simulink model "UAV_Model_template"  (R2025b)
settings: Solver=VariableStepAuto  StartTime=0.0  StopTime=50  FixedStep=Step_Size  RelTol=1e-3  EnableMultiTasking=on
values from neighbouring files (symbols this model uses):
  Init_Pos = [ 0.0, 0.0, -100.0 ]    [main_E2.m]
  Init_Rate = [ x_trim(4), x_trim(5), x_trim(6) ]    [main_E2.m]
  Init_Vel = [ x_trim(1), x_trim(2), x_trim(3) ]    [main_E2.m]
  K_p = 1    [model_data.mat]
  K_q = 3    [model_data.mat]
  K_r = -1    [model_data.mat]
  K_roll = 3    [model_data.mat]
  K_theta = 4    [model_data.mat]
  K_vt = 5    [model_data.mat]
  Max_del_a = 0.523598775598    [model_data.mat]
  Max_del_e = 0.523598775598    [model_data.mat]
  Max_del_r = 0.523598775598    [model_data.mat]
  Max_del_T = 10    [model_data.mat]
  tau_a = 0.5    [model_data.mat]
  tau_e = 0.5    [model_data.mat]
  tau_r = 0.5    [model_data.mat]
  tau_T = 0.2    [model_data.mat]
  u_trim = [0.186847387435 -0.168691706131 2.20732861993e-24 8.61178457979e-24]    [model_data.mat]
  UNIT_GRAV = 9.81    [main_E2.m]
  x_trim = [19.7714170486 1.55747135078e-22 3.01513977975 3.57452064707e-26 1.12807765409e-24 6.034407576e-27 1.79365250696e-25 0.151333968898 -1.40042455829e-45 -2.75841298622e-46 3.7376372575e-41 -5.9107417756e-40]    [model_data.mat]
libraries: UAV_Model_library x16, aerolibconvert2 x3, shared6dofsys x1, aerolibtransform2 x1, matrix_library x1, sharedutil x1, shared6dof x1
settings Model: Creator=e803534  LastModifiedBy=82104
settings SolverCC: AlgebraicLoopSolver=TrustRegion
settings DataIOCC: ReturnWorkspaceOutputs=off
settings OptimizationCC: LifeSpan=inf
settings DebuggingCC: UnconnectedInputMsg=warning  UnconnectedOutputMsg=warning  UnconnectedLineMsg=warning  SFUnexpectedBacktrackingDiag=warning  SFNoUnconditionalDefaultTransitionDiag=warning  ArithmeticOperatorsInVariantConditions=warning
settings ModelReferenceCC: EnableRefExpFcnMdlSchedulingChecks=on
settings SFSimCC: SimUseLocalCustomCode=off  CustomCodeUndefinedFunction=UseInterfaceOnly
settings RTWCC: RTWUseLocalCustomCode=off  GPUComputeCapability=3.5
settings CodeAppCC: StateflowObjectComments=on
settings GRTTargetCC: TargetLangStandard=C89/C90 (ANSI)
settings ConfigComp: CovMetricSettings=dw  CovSaveCumulativeToWorkspaceVar=on  CovSaveSingleToWorkspaceVar=on  CovExternalEMLEnable=off

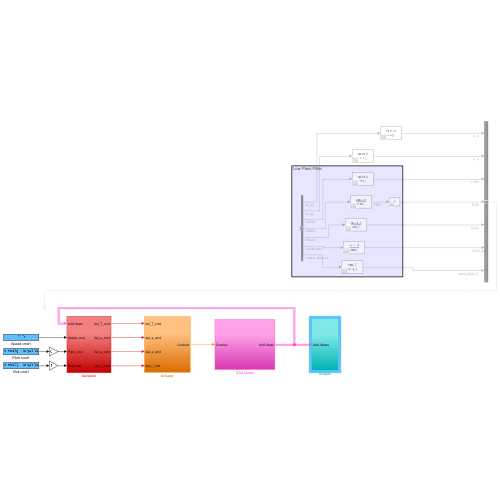
[thumbnail: Simulink's stored preview of the top-level diagram]
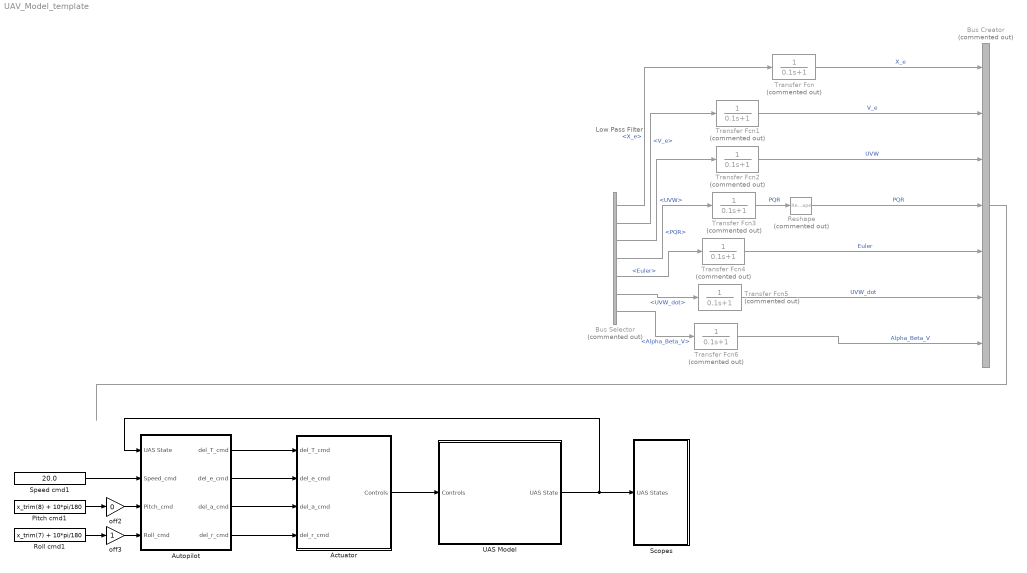
== system UAV_Model_template ==
  note: Low Pass Filter
  Actuator : Subsystem
  Autopilot : Subsystem
  Bus Creator : BusCreator  Commented=on  Inputs=7
  Bus Selector : BusSelector  Commented=on  OutputSignals=X_e,V_e,UVW,PQR,Euler,UVW_dot,Alpha_Beta_V
  Pitch cmd1 : Constant  Value=x_trim(8) + 10*pi/180
  Reshape : Reshape  Commented=on  OutputDimensionality=Customize  OutputDimensions=[3,1]
  Roll cmd1 : Constant  Value=x_trim(7) + 10*pi/180
  Scopes : Subsystem
  Speed cmd1 : Constant  Value=20.0
  Transfer Fcn{,1..6} (7 alike) : TransferFcn  Commented=on  Denominator=[0.1 1]
  UAS Model : Subsystem
  off2 : Gain  Gain=0
  off3 : Gain
  wires:
  Speed cmd1/1 -> Autopilot/2(Speed_cmd)
  Autopilot/1(del_T_cmd) -> Actuator/1(del_T_cmd)
  Autopilot/2(del_e_cmd) -> Actuator/2(del_e_cmd)
  Autopilot/4(del_r_cmd) -> Actuator/4(del_r_cmd)
  Autopilot/3(del_a_cmd) -> Actuator/3(del_a_cmd)
  off2/1 -> Autopilot/3(Pitch_cmd)
  Pitch cmd1/1 -> off2/1
  off3/1 -> Autopilot/4(Roll_cmd)
  Roll cmd1/1 -> off3/1
  UAS Model/1(UAS State) -> Autopilot/1(UAS State), Scopes/1(UAS States)
  Actuator/1(Controls) -> UAS Model/1(Controls)
  Bus Selector/1 -> Transfer Fcn/1  "<X_e>"
  Bus Selector/2 -> Transfer Fcn1/1  "<V_e>"
  Bus Selector/3 -> Transfer Fcn2/1  "<UVW>"
  Bus Selector/4 -> Transfer Fcn3/1  "<PQR>"
  Bus Selector/5 -> Transfer Fcn4/1  "<Euler>"
  Bus Selector/6 -> Transfer Fcn5/1  "<UVW_dot>"
  Bus Selector/7 -> Transfer Fcn6/1  "<Alpha_Beta_V>"
  Transfer Fcn/1 -> Bus Creator/1  "X_e"
  Reshape/1 -> Bus Creator/4  "PQR"
  Transfer Fcn1/1 -> Bus Creator/2  "V_e"
  Transfer Fcn5/1 -> Bus Creator/6  "UVW_dot"
  Transfer Fcn4/1 -> Bus Creator/5  "Euler"
  Transfer Fcn6/1 -> Bus Creator/7  "Alpha_Beta_V"
  Transfer Fcn2/1 -> Bus Creator/3  "UVW"
  Bus Creator/1 -> ?
  Transfer Fcn3/1 -> Reshape/1  "PQR"

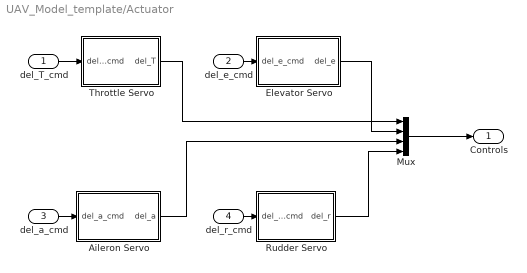
== system UAV_Model_template/Actuator ==
  del_T_cmd : Inport
  del_e_cmd : Inport  Port=2
  del_a_cmd : Inport  Port=3
  del_r_cmd : Inport  Port=4
  Aileron Servo : Subsystem
  Elevator Servo : Subsystem
  Mux : Mux
  Rudder Servo : Subsystem
  Throttle Servo : Subsystem
  Controls : Outport
  wires:
  del_T_cmd/1 -> Throttle Servo/1(del_T_cmd)
  del_r_cmd/1 -> Rudder Servo/1(del_r_cmd)
  del_a_cmd/1 -> Aileron Servo/1(del_a_cmd)
  del_e_cmd/1 -> Elevator Servo/1(del_e_cmd)
  Throttle Servo/1(del_T) -> Mux/1
  Elevator Servo/1(del_e) -> Mux/2
  Aileron Servo/1(del_a) -> Mux/3
  Rudder Servo/1(del_r) -> Mux/4
  Mux/1 -> Controls/1

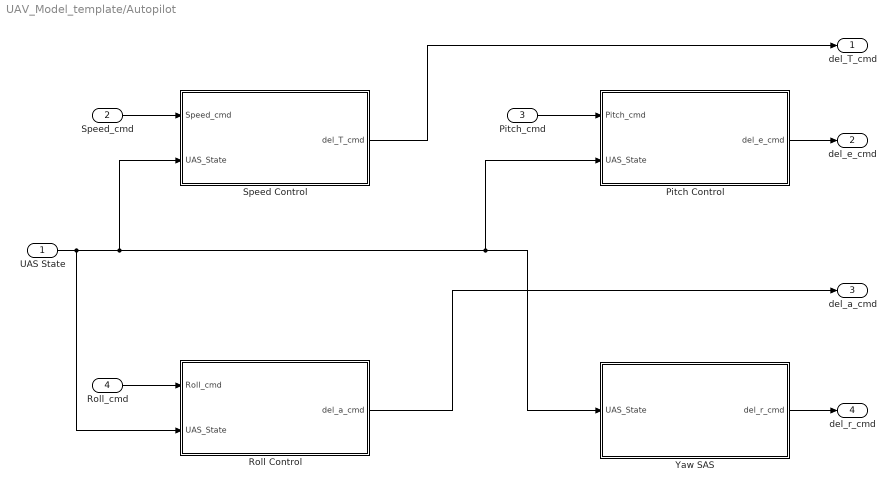
== system UAV_Model_template/Autopilot ==
  UAS State : Inport
  Speed_cmd : Inport  Port=2
  Pitch_cmd : Inport  Port=3
  Roll_cmd : Inport  Port=4
  Pitch Control : Subsystem
  Roll Control : Subsystem
  Speed Control : Subsystem
  Yaw SAS : Subsystem
  del_T_cmd : Outport
  del_e_cmd : Outport  Port=2
  del_a_cmd : Outport  Port=3
  del_r_cmd : Outport  Port=4
  wires:
  Speed_cmd/1 -> Speed Control/1(Speed_cmd)
  Roll_cmd/1 -> Roll Control/1(Roll_cmd)
  Pitch_cmd/1 -> Pitch Control/1(Pitch_cmd)
  Speed Control/1(del_T_cmd) -> del_T_cmd/1
  UAS State/1 -> Yaw SAS/1(UAS_State), Pitch Control/2(UAS_State), Speed Control/2(UAS_State), Roll Control/2(UAS_State)
  Roll Control/1(del_a_cmd) -> del_a_cmd/1
  Pitch Control/1(del_e_cmd) -> del_e_cmd/1
  Yaw SAS/1(del_r_cmd) -> del_r_cmd/1

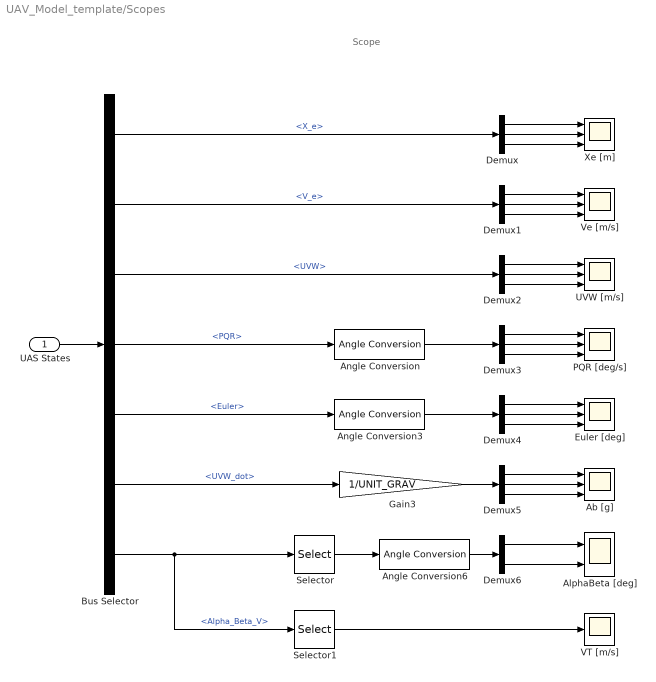
== system UAV_Model_template/Scopes ==
  note: Scope
  UAS States : Inport
  Ab [g] : Scope  NumInputPorts=3
      settings: ActiveDisplayYMinimum=-1  ActiveDisplayYMaximum=1  DataLoggingSaveFormat=Array
  AlphaBeta [deg] : Scope  NumInputPorts=2
      settings: ActiveDisplayYMinimum=6.34123  ActiveDisplayYMaximum=8.97339  DataLoggingVariableName=Xe15  DataLoggingSaveFormat=Array
  Angle Conversion : aerolibconvert2/Angle Conversion  IU=rad  OU=deg
  Angle Conversion3 : aerolibconvert2/Angle Conversion  IU=rad  OU=deg
  Angle Conversion6 : aerolibconvert2/Angle Conversion  IU=rad  OU=deg
  Bus Selector : BusSelector  OutputSignals=X_e,V_e,UVW,PQR,Euler,UVW_dot,Alpha_Beta_V
  Demux{,1..5} (6 alike) : Demux  Outputs=3
  Demux6 : Demux  Outputs=2
  Euler [deg] : Scope  NumInputPorts=3
      settings: ActiveDisplayYMinimum=-1.24407  ActiveDisplayYMaximum=11.19661  DataLoggingVariableName=Xe12  DataLoggingSaveFormat=Array
  Gain3 : Gain  Gain=1/UNIT_GRAV
  PQR [deg/s] : Scope  NumInputPorts=3
      settings: ActiveDisplayYMinimum=-1  ActiveDisplayYMaximum=1  DataLoggingVariableName=Xe9  DataLoggingSaveFormat=Array
  Selector : Selector  InputPortWidth=3  IndexOptions=Index vector (dialog)  Indices=[1 2]  OutputSizes=1
  Selector1 : Selector  InputPortWidth=3  IndexOptions=Index vector (dialog)  Indices=[3]  OutputSizes=1
  UVW [m/s] : Scope  NumInputPorts=3
      settings: ActiveDisplayYMinimum=19.747945965701106  ActiveDisplayYMaximum=19.982656794414307  DataLoggingVariableName=Xe6  DataLoggingSaveFormat=Array
  VT [m/s] : Scope
      settings: ActiveDisplayYMinimum=19.98074  ActiveDisplayYMaximum=20.17333  DataLoggingVariableName=Xe17  DataLoggingSaveFormat=Array
  Ve [m/s] : Scope  NumInputPorts=3
      settings: ActiveDisplayYMinimum=-24.908833461463328  ActiveDisplayYMaximum=25.058946482700829  DataLoggingVariableName=Xe3  DataLoggingSaveFormat=Array
  Xe [m] : Scope  NumInputPorts=3
      settings: ActiveDisplayYMinimum=-218.67892964413309  ActiveDisplayYMaximum=371.04226925636226  DataLoggingVariableName=Xe  DataLoggingSaveFormat=Array
  wires:
  UAS States/1 -> Bus Selector/1
  Bus Selector/1 -> Demux/1  "<X_e>"
  Bus Selector/2 -> Demux1/1  "<V_e>"
  Bus Selector/3 -> Demux2/1  "<UVW>"
  Bus Selector/4 -> Angle Conversion/1  "<PQR>"
  Bus Selector/5 -> Angle Conversion3/1  "<Euler>"
  Bus Selector/6 -> Gain3/1  "<UVW_dot>"
  Angle Conversion3/1 -> Demux4/1
  Angle Conversion/1 -> Demux3/1
  Selector1/1 -> VT [m/s]/1
  Gain3/1 -> Demux5/1
  Demux/1 -> Xe [m]/1
  Demux/2 -> Xe [m]/2
  Demux/3 -> Xe [m]/3
  Demux1/1 -> Ve [m/s]/1
  Demux1/2 -> Ve [m/s]/2
  Demux1/3 -> Ve [m/s]/3
  Demux2/1 -> UVW [m/s]/1
  Demux2/2 -> UVW [m/s]/2
  Demux2/3 -> UVW [m/s]/3
  Demux3/1 -> PQR [deg/s]/1
  Demux3/2 -> PQR [deg/s]/2
  Demux3/3 -> PQR [deg/s]/3
  Demux4/1 -> Euler [deg]/1
  Demux4/2 -> Euler [deg]/2
  Demux4/3 -> Euler [deg]/3
  Demux5/1 -> Ab [g]/1
  Demux5/2 -> Ab [g]/2
  Demux5/3 -> Ab [g]/3
  Demux6/2 -> AlphaBeta [deg]/2
  Demux6/1 -> AlphaBeta [deg]/1
  Angle Conversion6/1 -> Demux6/1
  Bus Selector/7 -> Selector1/1, Selector/1  "<Alpha_Beta_V>"
  Selector/1 -> Angle Conversion6/1

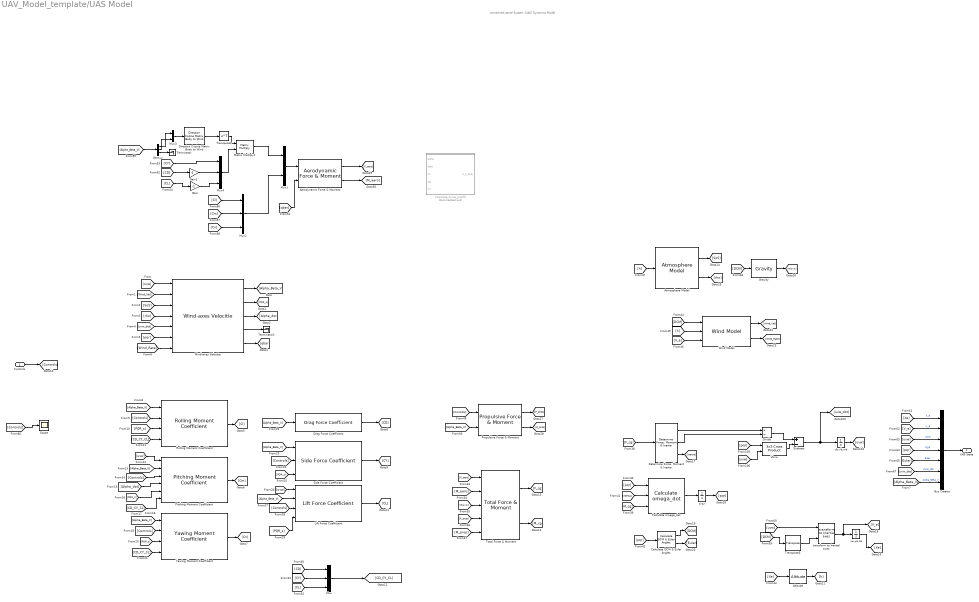
== system UAV_Model_template/UAS Model ==
  note: Unmanned Aerial System (UAS) Dynamics Model
  Controls : Inport
  Aerodynamic Force & Moment : UAV_Model_library/External Forces/Aerodynamics/Aerodynamic Force & Moment  SystemSampleTime=-1  VariantActivationTime=update diagram  EmptyChoice=off  PassThrough=off  PassThroughVariantControl=(default)  EmptyChoiceVariantControl=(default)  AllowFlexibleInterface=on  Latency=0  AutoFrameSizeCalculation=off
  Altitude : UAV_Model_library/Equations of Motion/Altitude  SystemSampleTime=-1  VariantActivationTime=update diagram  EmptyChoice=off  PassThrough=off  PassThroughVariantControl=(default)  EmptyChoiceVariantControl=(default)  AllowFlexibleInterface=on  Latency=0  AutoFrameSizeCalculation=off
  Atmosphere Model : UAV_Model_library/Envrionment/Atmosphere Model  SystemSampleTime=-1  VariantActivationTime=update diagram  EmptyChoice=off  PassThrough=off  PassThroughVariantControl=(default)  EmptyChoiceVariantControl=(default)  AllowFlexibleInterface=on  Latency=0  AutoFrameSizeCalculation=off
  Bus Creator : BusCreator  Inputs=7
  Calculate DCM & Euler Angles : UAV_Model_library/Equations of Motion/Calculate DCM & Euler Angles  SystemSampleTime=-1  VariantActivationTime=update diagram  EmptyChoice=off  PassThrough=off  PassThroughVariantControl=(default)  EmptyChoiceVariantControl=(default)  AllowFlexibleInterface=on  Latency=0  AutoFrameSizeCalculation=off
  Calculate omega_dot : shared6dofsys/Calculate omega_dot  aMode=aMode
  Calculate_Force_Coeffs : MATLAB Function  Commented=on  TreatAsAtomicUnit=on
  Demux : Demux  Outputs=3
  "Determine Force, Moment & Inertia" : UAV_Model_library/Equations of Motion/Determine Force, Moment & Inertia  SystemSampleTime=-1  VariantActivationTime=update diagram  EmptyChoice=off  PassThrough=off  PassThroughVariantControl=(default)  EmptyChoiceVariantControl=(default)  AllowFlexibleInterface=on  Latency=0  AutoFrameSizeCalculation=off
  Direction Cosine Matrix Body to Wind : aerolibtransform2/Direction Cosine Matrix Body to Wind
  Divide : Product  Inputs=*/
  Drag Force Coefficient : UAV_Model_library/External Forces/Aerodynamics/Aerodynamics coefficients/Drag Force Coefficient  SystemSampleTime=-1  VariantActivationTime=update diagram  EmptyChoice=off  PassThrough=off  PassThroughVariantControl=(default)  EmptyChoiceVariantControl=(default)  AllowFlexibleInterface=on  Latency=0  AutoFrameSizeCalculation=off
  Gain : Gain  Gain=-1
  Gain1 : Gain  Gain=-1
  Gravity : UAV_Model_library/Envrionment/Gravity  SystemSampleTime=-1  VariantActivationTime=update diagram  EmptyChoice=off  PassThrough=off  PassThroughVariantControl=(default)  EmptyChoiceVariantControl=(default)  AllowFlexibleInterface=on  Latency=0  AutoFrameSizeCalculation=off
  "Lift Force Coefficient  " : UAV_Model_library/External Forces/Aerodynamics/Aerodynamics coefficients/Lift Force Coefficient    SystemSampleTime=-1  VariantActivationTime=update diagram  EmptyChoice=off  PassThrough=off  PassThroughVariantControl=(default)  EmptyChoiceVariantControl=(default)  AllowFlexibleInterface=on  Latency=0  AutoFrameSizeCalculation=off
  Matrix Multiply1 : Product  Multiplication=Matrix(*)
  Mux : Mux  Inputs=3
  Mux1 : Mux  Inputs=2
  Mux2 : Mux  Inputs=3
  Mux3 : Mux  Inputs=2
  Mux4 : Mux  Inputs=3
  Pitching Moment Coefficient : UAV_Model_library/External Forces/Aerodynamics/Aerodynamics coefficients/Pitching Moment Coefficient  SystemSampleTime=-1  VariantActivationTime=update diagram  EmptyChoice=off  PassThrough=off  PassThroughVariantControl=(default)  EmptyChoiceVariantControl=(default)  AllowFlexibleInterface=on  Latency=0  AutoFrameSizeCalculation=off
  Propulsive Force & Moment : UAV_Model_library/External Forces/Propulsive/Propulsive Force & Moment  SystemSampleTime=-1  VariantActivationTime=update diagram  EmptyChoice=off  PassThrough=off  PassThroughVariantControl=(default)  EmptyChoiceVariantControl=(default)  AllowFlexibleInterface=on  Latency=0  AutoFrameSizeCalculation=off
  Rolling Moment Coefficient : UAV_Model_library/External Forces/Aerodynamics/Aerodynamics coefficients/Rolling Moment Coefficient  SystemSampleTime=-1  VariantActivationTime=update diagram  EmptyChoice=off  PassThrough=off  PassThroughVariantControl=(default)  EmptyChoiceVariantControl=(default)  AllowFlexibleInterface=on  Latency=0  AutoFrameSizeCalculation=off
  Scope : Scope
      settings: ActiveDisplayYMinimum=-2.6710074765417144  ActiveDisplayYMaximum=5.4030514529656211
  "Side Force Coefficient " : UAV_Model_library/External Forces/Aerodynamics/Aerodynamics coefficients/Side Force Coefficient   SystemSampleTime=-1  VariantActivationTime=update diagram  EmptyChoice=off  PassThrough=off  PassThroughVariantControl=(default)  EmptyChoiceVariantControl=(default)  AllowFlexibleInterface=on  Latency=0  AutoFrameSizeCalculation=off
  Subtract : Sum  Inputs=+-
  Terminator : Terminator
  Terminator1 : Terminator
  Total Force & Moment : UAV_Model_library/External Forces/Total Force & Moment  SystemSampleTime=-1  VariantActivationTime=update diagram  EmptyChoice=off  PassThrough=off  PassThroughVariantControl=(default)  EmptyChoiceVariantControl=(default)  AllowFlexibleInterface=on  Latency=0  AutoFrameSizeCalculation=off
  Transpose1 : Math  Operator=transpose
  Transpose3 : matrix_library/Transpose
  Vbxw : sharedutil/3x3 Cross Product  aMode=aMode
  Wind Model : UAV_Model_library/Envrionment/Wind Model  SystemSampleTime=-1  VariantActivationTime=update diagram  EmptyChoice=off  PassThrough=off  PassThroughVariantControl=(default)  EmptyChoiceVariantControl=(default)  AllowFlexibleInterface=on  Latency=0  AutoFrameSizeCalculation=off
  Wind-axes Velocitie : UAV_Model_library/External Forces/Aerodynamics/Wind-axes Velocitie  SystemSampleTime=-1  VariantActivationTime=update diagram  EmptyChoice=off  PassThrough=off  PassThroughVariantControl=(default)  EmptyChoiceVariantControl=(default)  AllowFlexibleInterface=on  Latency=0  AutoFrameSizeCalculation=off
  Yawing Moment Coefficient : UAV_Model_library/External Forces/Aerodynamics/Aerodynamics coefficients/Yawing Moment Coefficient  SystemSampleTime=-1  VariantActivationTime=update diagram  EmptyChoice=off  PassThrough=off  PassThroughVariantControl=(default)  EmptyChoiceVariantControl=(default)  AllowFlexibleInterface=on  Latency=0  AutoFrameSizeCalculation=off
  "p,q,r " : Integrator  InitialCondition=Init_Rate
  "transform to Inertial axes " : shared6dof/6DOF (Euler Angles)/transform to Inertial axes   SystemSampleTime=-1  VariantActivationTime=update diagram  EmptyChoice=off  PassThrough=off  PassThroughVariantControl=(default)  EmptyChoiceVariantControl=(default)  AllowFlexibleInterface=on  Latency=0  AutoFrameSizeCalculation=off
  ub,vb,wb : Integrator  InitialCondition=Init_Vel
  xe,ye,ze : Integrator  InitialCondition=Init_Pos
  UAS State : Outport  VectorParamsAs1DForOutWhenUnconnected=off
  wires:
  Controls/1 -> [Controls]
  [V_e] -> Bus Creator/2  "V_e"
  Bus Creator/1 -> UAS State/1
  [uvw_dot] -> Bus Creator/6  "UVW_dot"
  [Euler] -> Bus Creator/5  "Euler"
  [Xe] -> Bus Creator/1  "X_e"
  [uvw] -> Bus Creator/3  "UVW"
  [pqr] -> Bus Creator/4  "PQR"
  [uvw] -> Wind-axes Velocitie/1
  [Wind_Vel] -> Wind-axes Velocitie/2
  [SoS] -> Wind-axes Velocitie/3
  [rho] -> Wind-axes Velocitie/4
  [uvw_dot] -> Wind-axes Velocitie/5
  [pqr] -> Wind-axes Velocitie/6
  [Wind_Rate] -> Wind-axes Velocitie/7
  [Alpha_Beta_V] -> Bus Creator/7  "Alpha_Beta_V"
  Wind-axes Velocitie/1 -> [Alpha_Beta_V]
  Wind-axes Velocitie/2 -> [PQR_s]
  Wind-axes Velocitie/3 -> [Alpha_dot]
  Wind-axes Velocitie/4 -> Terminator1/1
  Wind-axes Velocitie/5 -> [qbar]
  [CD_CY_CL] -> Rolling Moment Coefficient/4
  [Controls] -> Rolling Moment Coefficient/2
  [PQR_s] -> Rolling Moment Coefficient/3
  [Alpha_Beta_V] -> Rolling Moment Coefficient/1
  Rolling Moment Coefficient/1 -> [Cl]
  [Alpha_Beta_V] -> Pitching Moment Coefficient/2
  [uvw] -> Pitching Moment Coefficient/1
  [Controls] -> Pitching Moment Coefficient/3
  [Alpha_dot] -> Pitching Moment Coefficient/4
  [PQR_s] -> Pitching Moment Coefficient/5
  [CD_CY_CL] -> Pitching Moment Coefficient/6
  Pitching Moment Coefficient/1 -> [Cm]
  [Alpha_Beta_V] -> Yawing Moment Coefficient/1
  [Controls] -> Yawing Moment Coefficient/2
  [PQR_s] -> Yawing Moment Coefficient/3
  [CD_CY_CL] -> Yawing Moment Coefficient/4
  Yawing Moment Coefficient/1 -> [Cn]
  [Alpha_Beta_V] -> Drag Force Coefficient/1
  [Alpha_Beta_V] -> "Side Force Coefficient "/1
  [Controls] -> "Side Force Coefficient "/2
  [PQR_s] -> "Side Force Coefficient "/3
  [uvw] -> "Lift Force Coefficient  "/1
  [Alpha_Beta_V] -> "Lift Force Coefficient  "/2
  [Controls] -> "Lift Force Coefficient  "/3
  [PQR_s] -> "Lift Force Coefficient  "/4
  "Lift Force Coefficient  "/1 -> [CL]
  "Side Force Coefficient "/1 -> [CY]
  Drag Force Coefficient/1 -> [CD]
  [CD] -> Mux/1
  [CY] -> Mux/2
  [CL] -> Mux/3
  Mux/1 -> [CD_CY_CL]
  [F_aero] -> Total Force & Moment/1
  [M_aero] -> Total Force & Moment/2
  [Gravity] -> Total Force & Moment/3
  [F_prop] -> Total Force & Moment/4
  [M_prop] -> Total Force & Moment/5
  Total Force & Moment/1 -> [F_cg]
  Total Force & Moment/2 -> [M_cg]
  [F_cg] -> "Determine Force, Moment & Inertia"/1
  [M_cg] -> Calculate omega_dot/3
  "Determine Force, Moment & Inertia"/3 -> [inertia]
  [pqr] -> Calculate omega_dot/1
  [inertia] -> Calculate omega_dot/2
  Calculate omega_dot/1 -> "p,q,r "/1
  "p,q,r "/1 -> [pqr]
  [pqr] -> Calculate DCM & Euler Angles/1
  Calculate DCM & Euler Angles/1 -> [DCM]
  Calculate DCM & Euler Angles/2 -> [Euler]
  [DCM] -> Wind Model/1
  [h] -> Wind Model/2
  [V_e] -> Wind Model/3
  Wind Model/1 -> [Wind_Vel]
  Wind Model/2 -> [Wind_Rate]
  [h] -> Atmosphere Model/1
  Atmosphere Model/1 -> [SoS]
  Atmosphere Model/2 -> [rho]
  [DCM] -> Gravity/1
  Gravity/1 -> [Gravity]
  [Controls] -> Propulsive Force & Moment/1
  [Alpha_Beta_V] -> Propulsive Force & Moment/2
  Propulsive Force & Moment/1 -> [F_prop]
  Propulsive Force & Moment/2 -> [M_prop]
  Aerodynamic Force & Moment/2 -> [M_aero]
  Aerodynamic Force & Moment/1 -> [F_aero]
  [qbar] -> Aerodynamic Force & Moment/2
  [CL] -> Gain/1
  [Alpha_Beta_V] -> Demux/1
  Demux/3 -> Terminator/1
  Matrix Multiply1/1 -> Mux1/1
  [Cl] -> Mux2/1
  [Cm] -> Mux2/2
  [Cn] -> Mux2/3
  Mux2/1 -> Mux1/2
  Mux1/1 -> Aerodynamic Force & Moment/1
  [pqr] -> Vbxw/1
  "Determine Force, Moment & Inertia"/2 -> Divide/2
  ub,vb,wb/1 -> [uvw]
  Altitude/1 -> [h]
  [Xe] -> Altitude/1
  [uvw] -> Vbxw/2
  Vbxw/1 -> Subtract/2
  Divide/1 -> Subtract/1
  Subtract/1 -> [uvw_dot], ub,vb,wb/1
  "Determine Force, Moment & Inertia"/1 -> Divide/1
  Demux/1 -> Mux3/1
  Demux/2 -> Mux3/2
  [CD] -> Gain1/1
  [CY] -> Mux4/1
  Gain1/1 -> Mux4/2
  Gain/1 -> Mux4/3
  Mux4/1 -> Matrix Multiply1/2
  [uvw] -> "transform to Inertial axes "/1
  [DCM] -> Transpose3/1
  Transpose3/1 -> "transform to Inertial axes "/2
  xe,ye,ze/1 -> [Xe]
  "transform to Inertial axes "/1 -> xe,ye,ze/1, [V_e]
  [Controls] -> Scope/1
  Mux3/1 -> Direction Cosine Matrix Body to Wind/1
  Direction Cosine Matrix Body to Wind/1 -> Transpose1/1
  Transpose1/1 -> Matrix Multiply1/1

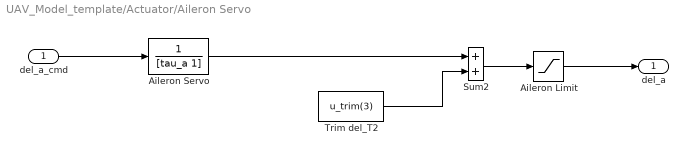
== system UAV_Model_template/Actuator/Aileron Servo ==
  del_a_cmd : Inport
  Aileron Limit : Saturate  UpperLimit=Max_del_a  LowerLimit=-Max_del_a
  Aileron Servo : TransferFcn  Denominator=[tau_a 1]
  Sum2 : Sum  SaturateOnIntegerOverflow=on
  Trim del_T2 : Constant  Value=u_trim(3)
  del_a : Outport  VectorParamsAs1DForOutWhenUnconnected=off
  wires:
  Trim del_T2/1 -> Sum2/2
  Sum2/1 -> Aileron Limit/1
  del_a_cmd/1 -> Aileron Servo/1
  Aileron Servo/1 -> Sum2/1
  Aileron Limit/1 -> del_a/1

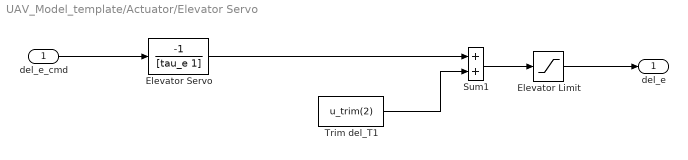
== system UAV_Model_template/Actuator/Elevator Servo ==
  del_e_cmd : Inport
  Elevator Limit : Saturate  UpperLimit=Max_del_e  LowerLimit=-Max_del_e
  Elevator Servo : TransferFcn  Numerator=[-1]  Denominator=[tau_e 1]
  Sum1 : Sum  SaturateOnIntegerOverflow=on
  Trim del_T1 : Constant  Value=u_trim(2)
  del_e : Outport  VectorParamsAs1DForOutWhenUnconnected=off
  wires:
  Sum1/1 -> Elevator Limit/1
  del_e_cmd/1 -> Elevator Servo/1
  Trim del_T1/1 -> Sum1/2
  Elevator Servo/1 -> Sum1/1
  Elevator Limit/1 -> del_e/1

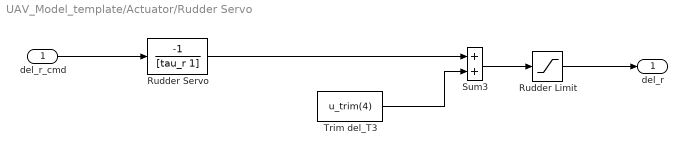
== system UAV_Model_template/Actuator/Rudder Servo ==
  del_r_cmd : Inport
  Rudder Limit : Saturate  UpperLimit=Max_del_r  LowerLimit=-Max_del_r
  Rudder Servo : TransferFcn  Numerator=[-1]  Denominator=[tau_r 1]
  Sum3 : Sum  SaturateOnIntegerOverflow=on
  Trim del_T3 : Constant  Value=u_trim(4)
  del_r : Outport  VectorParamsAs1DForOutWhenUnconnected=off
  wires:
  Trim del_T3/1 -> Sum3/2
  Rudder Limit/1 -> del_r/1
  Rudder Servo/1 -> Sum3/1
  del_r_cmd/1 -> Rudder Servo/1
  Sum3/1 -> Rudder Limit/1

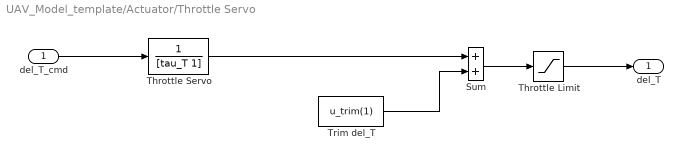
== system UAV_Model_template/Actuator/Throttle Servo ==
  del_T_cmd : Inport
  Sum : Sum  SaturateOnIntegerOverflow=on
  Throttle Limit : Saturate  UpperLimit=Max_del_T  LowerLimit=-Max_del_T
  Throttle Servo : TransferFcn  Denominator=[tau_T 1]
  Trim del_T : Constant  Value=u_trim(1)
  del_T : Outport  VectorParamsAs1DForOutWhenUnconnected=off
  wires:
  del_T_cmd/1 -> Throttle Servo/1
  Sum/1 -> Throttle Limit/1
  Throttle Servo/1 -> Sum/1
  Trim del_T/1 -> Sum/2
  Throttle Limit/1 -> del_T/1

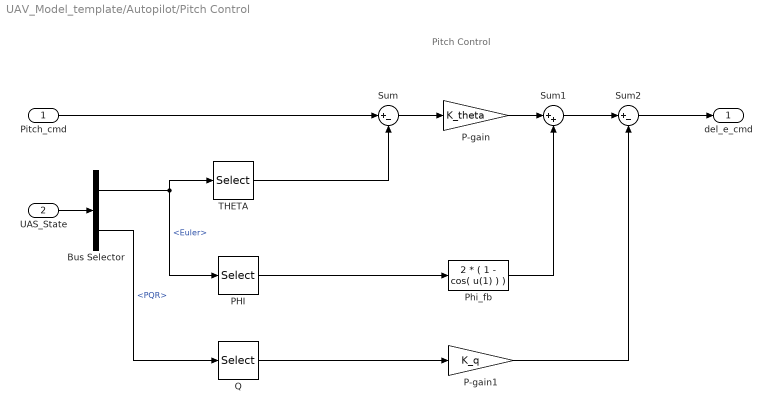
== system UAV_Model_template/Autopilot/Pitch Control ==
  note: Pitch Control
  Pitch_cmd : Inport
  UAS_State : Inport  Port=2
  Bus Selector : BusSelector  OutputSignals=Euler,PQR
  P-gain : Gain  Gain=K_theta
  P-gain1 : Gain  Gain=K_q
  PHI : Selector  InputPortWidth=3  IndexOptions=Index vector (dialog)  Indices=[1]  OutputSizes=1
  Phi_fb : Fcn  Expr=2 * ( 1 - cos( u(1) ) )
  Q : Selector  InputPortWidth=3  IndexOptions=Index vector (dialog)  Indices=[2]  OutputSizes=1
  Sum : Sum  Inputs=|+-
  Sum1 : Sum  Inputs=|++
  Sum2 : Sum  Inputs=|+-
  THETA : Selector  InputPortWidth=3  IndexOptions=Index vector (dialog)  Indices=[2]  OutputSizes=1
  del_e_cmd : Outport  VectorParamsAs1DForOutWhenUnconnected=off
  wires:
  Pitch_cmd/1 -> Sum/1
  Sum/1 -> P-gain/1
  THETA/1 -> Sum/2
  P-gain/1 -> Sum1/1
  Q/1 -> P-gain1/1
  PHI/1 -> Phi_fb/1
  Phi_fb/1 -> Sum1/2
  Sum1/1 -> Sum2/1
  P-gain1/1 -> Sum2/2
  Sum2/1 -> del_e_cmd/1
  Bus Selector/1 -> THETA/1, PHI/1  "<Euler>"
  UAS_State/1 -> Bus Selector/1
  Bus Selector/2 -> Q/1  "<PQR>"

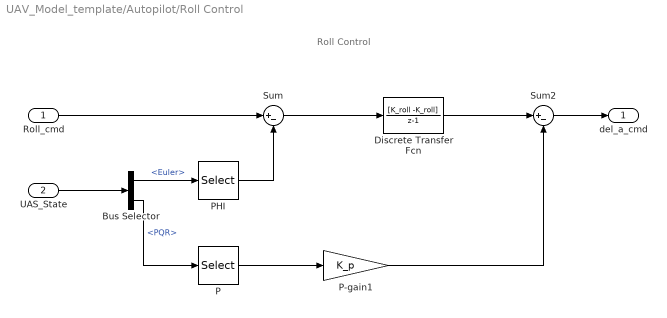
== system UAV_Model_template/Autopilot/Roll Control ==
  note: Roll Control
  Roll_cmd : Inport
  UAS_State : Inport  Port=2
  Bus Selector : BusSelector  OutputSignals=Euler,PQR
  Discrete Transfer Fcn : DiscreteTransferFcn  Numerator=[K_roll -K_roll]  Denominator=[1 -1]
  P : Selector  InputPortWidth=3  IndexOptions=Index vector (dialog)  Indices=[1]  OutputSizes=1
  P-gain1 : Gain  Gain=K_p
  PHI : Selector  InputPortWidth=3  IndexOptions=Index vector (dialog)  Indices=[1]  OutputSizes=1
  Sum : Sum  Inputs=|+-
  Sum2 : Sum  Inputs=|+-
  del_a_cmd : Outport  VectorParamsAs1DForOutWhenUnconnected=off
  wires:
  Sum2/1 -> del_a_cmd/1
  P-gain1/1 -> Sum2/2
  Discrete Transfer Fcn/1 -> Sum2/1
  P/1 -> P-gain1/1
  Sum/1 -> Discrete Transfer Fcn/1
  Roll_cmd/1 -> Sum/1
  PHI/1 -> Sum/2
  UAS_State/1 -> Bus Selector/1
  Bus Selector/1 -> PHI/1  "<Euler>"
  Bus Selector/2 -> P/1  "<PQR>"

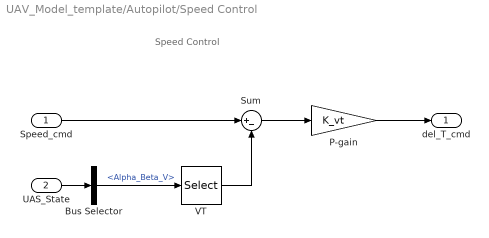
== system UAV_Model_template/Autopilot/Speed Control ==
  note: Speed Control
  Speed_cmd : Inport
  UAS_State : Inport  Port=2
  Bus Selector : BusSelector  OutputSignals=Alpha_Beta_V
  P-gain : Gain  Gain=K_vt
  Sum : Sum  Inputs=|+-
  VT : Selector  InputPortWidth=3  IndexOptions=Index vector (dialog)  Indices=[3]  OutputSizes=1
  del_T_cmd : Outport  VectorParamsAs1DForOutWhenUnconnected=off
  wires:
  P-gain/1 -> del_T_cmd/1
  UAS_State/1 -> Bus Selector/1
  VT/1 -> Sum/2
  Sum/1 -> P-gain/1
  Speed_cmd/1 -> Sum/1
  Bus Selector/1 -> VT/1  "<Alpha_Beta_V>"

== system UAV_Model_template/Autopilot/Yaw SAS ==
  note: Yaw SAS (Stability Augmented System)
  UAS_State : Inport
  Bus Selector : BusSelector  OutputSignals=PQR
  P-gain1 : Gain  Gain=K_r
  R : Selector  InputPortWidth=3  IndexOptions=Index vector (dialog)  Indices=[3]  OutputSizes=1
  del_r_cmd : Outport  VectorParamsAs1DForOutWhenUnconnected=off
  wires:
  UAS_State/1 -> Bus Selector/1
  R/1 -> P-gain1/1
  P-gain1/1 -> del_r_cmd/1
  Bus Selector/1 -> R/1  "<PQR>"

== matlab function UAV_Model_template/UAS Model/Calculate_Force_Coeffs ==
  data: alpha input; C_F_body output; beta input; CL input; CD input; CY input
function C_F_body  = Calculate_Force_Coeffs(alpha, beta, CL, CD, CY)

ca = cos(alpha);
sa = sin(alpha);
cb = cos(beta);
sb = sin(beta);

C_wb = [ ca*cb, -ca*sb, -sa;
         sb   ,  cb   ,  0;
         sa*cb, -sa*sb,  ca ];

C_F_wind = [-CD; CY; -CL];

C_F_body = C_wb * C_F_wind;

end
